simulink model "Form_Finding_Simulink"  (R2022a)
settings: Solver=ode14x  StartTime=0.0  StopTime=0.2  FixedStep=0.00005  RelTol=1e-3
values from neighbouring files (symbols this model uses):
  a_joint = 160/180*pi    (= 2.79252680319)    [Form_Finding_Activation.m]
  F_motor = F    (= 0)    [Form_Finding_Activation.m]
  g = [0;0;-9.81]    [Form_Finding_Activation.m]
  k_cable = 1200    [Form_Finding_Activation.m]
  k_joint = 35    [Form_Finding_Activation.m]
  l_cable = sqrt(6)/4*l_leg*sin(a_joint/2)*(1 - delta)    [Form_Finding_Activation.m]
  m_bar = density*(l_leg*pi*0.005^2)+ m_motor + m_battery    (= 0.662767695314)    [Form_Finding_Activation.m]
  x10_ini = x4_ini+[0 -2*bent_bar 0]    [Form_Finding_Activation.m]
  x11_ini = 2*bent_bar*rotVec([1 0 0],[0 1 0],-90-theta) + x5_ini    [Form_Finding_Activation.m]
  x12_ini = 2*bent_bar*rotVec([1 0 0],[0 1 0],-theta) + x6_ini    [Form_Finding_Activation.m]
  x1_ini = [0 0 0]    [Form_Finding_Activation.m]
  x2_ini = bent_bar*rotVec([1 0 0],[0 1 0],-theta)+ 0.5*sep*rotVec([1 0 0],[0 1 0],90-theta) + [0 sep/2 0]    [Form_Finding_Activation.m]
  x3_ini = [d6x   -sep/2         0]    [Form_Finding_Activation.m]
  x4_ini = bent_bar*rotVec([1 0 0],[0 1 0],-theta) + 0.5*sep*rotVec([1 0 0],[0 1 0],-90-theta) + [0 sep/2 0]    [Form_Finding_Activation.m]
  x5_ini = sep*rotVec([1 0 0],[0 1 0],-theta) + x3_ini    [Form_Finding_Activation.m]
  x6_ini = [0 -sep 0]    [Form_Finding_Activation.m]
  x7_ini = 2*bent_bar*rotVec([1 0 0],[0 1 0],-theta) + x1_ini    [Form_Finding_Activation.m]
  x8_ini = x2_ini + [0 -2*bent_bar 0]    [Form_Finding_Activation.m]
  x9_ini = 2*bent_bar*rotVec([1 0 0],[0 1 0],-90-theta) + x3_ini    [Form_Finding_Activation.m]
undefined symbols (not defined in the file or in its folder): l_bar
(part 1 of 2)
settings Model: Creator=LZY-ALIENWARE15  LastModifiedBy=S2974177
settings SolverCC: ExtrapolationOrder=3  AlgebraicLoopSolver=TrustRegion
settings DebuggingCC: UnconnectedInputMsg=warning  UnconnectedOutputMsg=warning  UnconnectedLineMsg=warning  SFMachineParentedDataDiag=warning
settings RTWCC: DLArmComputeVersion=19.05

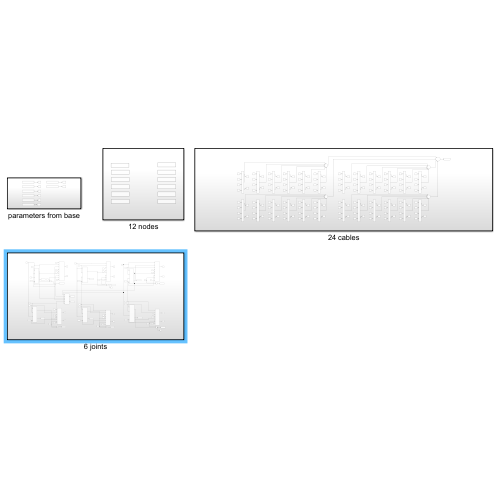
[thumbnail: Simulink's stored preview of the top-level diagram]
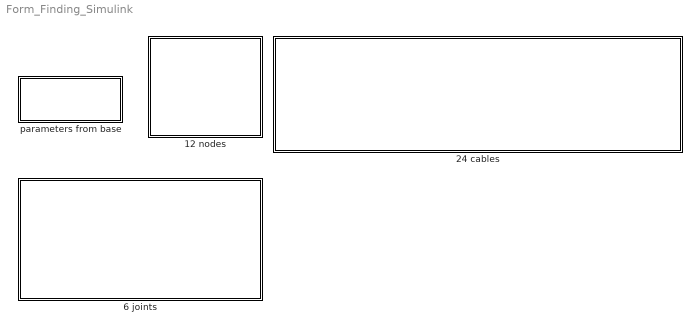
== system Form_Finding_Simulink ==
  "12 nodes " : Subsystem
  24 cables : Subsystem
  6 joints : Subsystem
  parameters from base : Subsystem

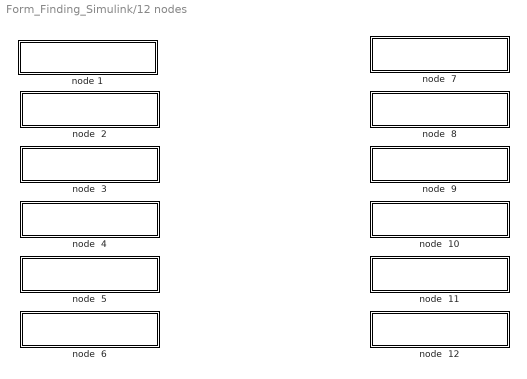
== system Form_Finding_Simulink/12 nodes  ==
  node  10 : Subsystem
  node  11 : Subsystem
  node  12 : Subsystem
  node  2 : Subsystem
  node  3 : Subsystem
  node  4 : Subsystem
  node  5 : Subsystem
  node  6 : Subsystem
  node  7 : Subsystem
  node  8 : Subsystem
  node  9 : Subsystem
  node 1 : Subsystem

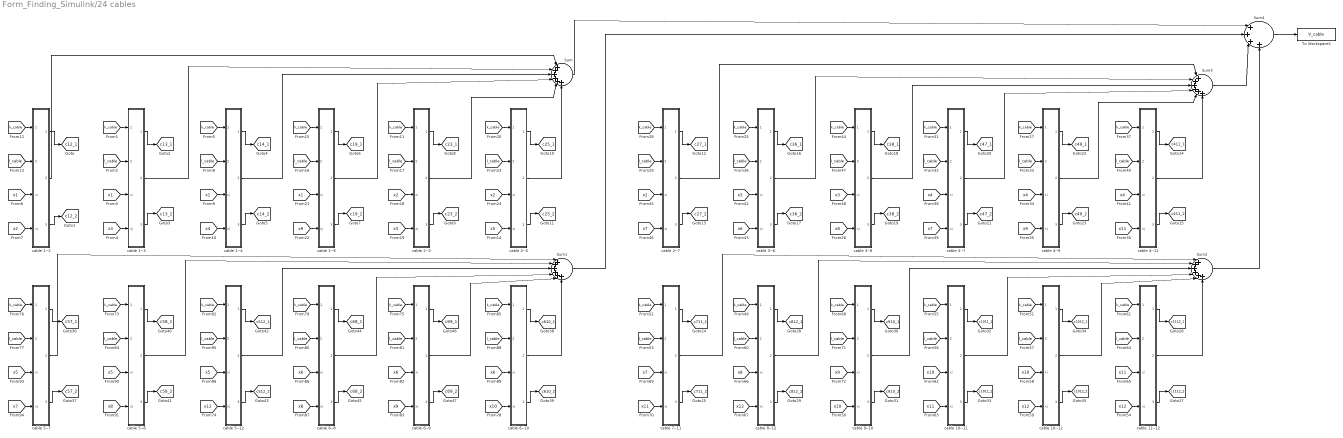
== system Form_Finding_Simulink/24 cables ==
  Sum{,1..3} (4 alike) : Sum  Inputs=|++++++
  Sum4 : Sum  Inputs=|++++
  To Workspace1 : ToWorkspace  VariableName=V_cable  SaveFormat=Timeseries  SampleTime=-1
  cable 1--2 : MATLAB Function  TreatAsAtomicUnit=on
  cable 1--3 : MATLAB Function  TreatAsAtomicUnit=on
  cable 1--4 : MATLAB Function  TreatAsAtomicUnit=on
  cable 1--9 : MATLAB Function  TreatAsAtomicUnit=on
  cable 10--11 : MATLAB Function  TreatAsAtomicUnit=on
  cable 10--12 : MATLAB Function  TreatAsAtomicUnit=on
  cable 11--12 : MATLAB Function  TreatAsAtomicUnit=on
  cable 2--3 : MATLAB Function  TreatAsAtomicUnit=on
  cable 2--5 : MATLAB Function  TreatAsAtomicUnit=on
  cable 2--7 : MATLAB Function  TreatAsAtomicUnit=on
  cable 3--6 : MATLAB Function  TreatAsAtomicUnit=on
  cable 3--8 : MATLAB Function  TreatAsAtomicUnit=on
  cable 4--11 : MATLAB Function  TreatAsAtomicUnit=on
  cable 4--7 : MATLAB Function  TreatAsAtomicUnit=on
  cable 4--9 : MATLAB Function  TreatAsAtomicUnit=on
  cable 5--12 : MATLAB Function  TreatAsAtomicUnit=on
  cable 5--7 : MATLAB Function  TreatAsAtomicUnit=on
  cable 5--8 : MATLAB Function  TreatAsAtomicUnit=on
  cable 6--10 : MATLAB Function  TreatAsAtomicUnit=on
  cable 6--8 : MATLAB Function  TreatAsAtomicUnit=on
  cable 6--9 : MATLAB Function  TreatAsAtomicUnit=on
  cable 7--11 : MATLAB Function  TreatAsAtomicUnit=on
  cable 8--12 : MATLAB Function  TreatAsAtomicUnit=on
  cable 9--10 : MATLAB Function  TreatAsAtomicUnit=on
  tag scope: c1011_1=global, c1011_2=global, c1012_1=global, c1012_2=global, c1112_1=global, c1112_2=global, c12_1=global, c12_2=global, c13_1=global, c13_2=global, c14_1=global, c14_2=global, c19_1=global, c19_2=global, c23_1=global, c23_2=global, c25_1=global, c25_2=global, c27_1=global, c27_2=global, c36_1=global, c36_2=global, c38_1=global, c38_2=global, c411_1=global, c411_2=global, c47_1=global, c47_2=global, c49_1=global, c49_2=global, c512_1=global, c512_2=global, c57_1=global, c57_2=global, c58_1=global, c58_2=global, c610_1=global, c610_2=global, c68_1=global, c68_2=global, c69_1=global, c69_2=global, c711_1=global, c711_2=global, c812_1=global, c812_2=global, c910_1=global, c910_2=global
  wires:
  [k_cable] -> cable 1--2/1(k_cable)
  [x1] -> cable 1--2/3(xi)
  [x2] -> cable 1--2/4(xj)
  cable 1--2/1(out_i) -> [c12_1]
  cable 1--2/3(out_j) -> [c12_2]
  [l_cable] -> cable 1--2/2(l_cable)
  [l_cable] -> cable 1--3/2(l_cable)
  [x1] -> cable 1--3/3(xi)
  [x3] -> cable 1--3/4(xj)
  cable 1--3/3(out_j) -> [c13_2]
  [k_cable] -> cable 1--3/1(k_cable)
  cable 1--3/1(out_i) -> [c13_1]
  [l_cable] -> cable 1--4/2(l_cable)
  [x1] -> cable 1--4/3(xi)
  [x4] -> cable 1--4/4(xj)
  cable 1--4/3(out_j) -> [c14_2]
  [k_cable] -> cable 1--4/1(k_cable)
  cable 1--4/1(out_i) -> [c14_1]
  [l_cable] -> cable 2--3/2(l_cable)
  [k_cable] -> cable 2--5/1(k_cable)
  cable 2--5/1(out_i) -> [c25_1]
  [x2] -> cable 2--5/3(xi)
  cable 2--5/3(out_j) -> [c25_2]
  cable 2--3/1(out_i) -> [c23_1]
  cable 2--3/3(out_j) -> [c23_2]
  [x3] -> cable 2--3/4(xj)
  [x1] -> cable 1--9/3(xi)
  [l_cable] -> cable 1--9/2(l_cable)
  [l_cable] -> cable 2--5/2(l_cable)
  [x9] -> cable 1--9/4(xj)
  [k_cable] -> cable 1--9/1(k_cable)
  [x2] -> cable 2--3/3(xi)
  cable 1--9/3(out_j) -> [c19_2]
  [k_cable] -> cable 2--3/1(k_cable)
  cable 1--9/1(out_i) -> [c19_1]
  [x5] -> cable 2--5/4(xj)
  [l_cable] -> cable 3--6/2(l_cable)
  [k_cable] -> cable 3--8/1(k_cable)
  cable 3--8/1(out_i) -> [c38_1]
  cable 3--8/3(out_j) -> [c38_2]
  cable 3--6/1(out_i) -> [c36_1]
  cable 3--6/3(out_j) -> [c36_2]
  [x6] -> cable 3--6/4(xj)
  [x7] -> cable 4--7/4(xj)
  [l_cable] -> cable 4--7/2(l_cable)
  [x4] -> cable 4--7/3(xi)
  [x9] -> cable 4--9/4(xj)
  cable 4--9/3(out_j) -> [c49_2]
  cable 4--11/3(out_j) -> [c411_2]
  [x4] -> cable 4--11/3(xi)
  [x11] -> cable 4--11/4(xj)
  cable 4--9/1(out_i) -> [c49_1]
  cable 4--7/1(out_i) -> [c47_1]
  [k_cable] -> cable 4--9/1(k_cable)
  cable 4--7/3(out_j) -> [c47_2]
  [k_cable] -> cable 4--7/1(k_cable)
  [x4] -> cable 4--9/3(xi)
  [x7] -> cable 2--7/4(xj)
  cable 2--7/3(out_j) -> [c27_2]
  [x3] -> cable 3--6/3(xi)
  [k_cable] -> cable 2--7/1(k_cable)
  [l_cable] -> cable 4--11/2(l_cable)
  cable 4--11/1(out_i) -> [c411_1]
  [x3] -> cable 3--8/3(xi)
  cable 2--7/1(out_i) -> [c27_1]
  [k_cable] -> cable 3--6/1(k_cable)
  [x8] -> cable 3--8/4(xj)
  [k_cable] -> cable 4--11/1(k_cable)
  [x2] -> cable 2--7/3(xi)
  [l_cable] -> cable 2--7/2(l_cable)
  [l_cable] -> cable 3--8/2(l_cable)
  [l_cable] -> cable 4--9/2(l_cable)
  [l_cable] -> cable 8--12/2(l_cable)
  [k_cable] -> cable 9--10/1(k_cable)
  cable 9--10/1(out_i) -> [c910_1]
  cable 9--10/3(out_j) -> [c910_2]
  cable 8--12/1(out_i) -> [c812_1]
  cable 8--12/3(out_j) -> [c812_2]
  [x12] -> cable 8--12/4(xj)
  [x11] -> cable 10--11/4(xj)
  [l_cable] -> cable 10--11/2(l_cable)
  [x10] -> cable 10--11/3(xi)
  [x12] -> cable 10--12/4(xj)
  cable 10--12/3(out_j) -> [c1012_2]
  cable 11--12/3(out_j) -> [c1112_2]
  [x11] -> cable 11--12/3(xi)
  [x12] -> cable 11--12/4(xj)
  cable 10--12/1(out_i) -> [c1012_1]
  cable 10--11/1(out_i) -> [c1011_1]
  [k_cable] -> cable 10--12/1(k_cable)
  cable 10--11/3(out_j) -> [c1011_2]
  [k_cable] -> cable 10--11/1(k_cable)
  [x10] -> cable 10--12/3(xi)
  [x11] -> cable 7--11/4(xj)
  cable 7--11/3(out_j) -> [c711_2]
  [x8] -> cable 8--12/3(xi)
  [k_cable] -> cable 7--11/1(k_cable)
  [l_cable] -> cable 11--12/2(l_cable)
  cable 11--12/1(out_i) -> [c1112_1]
  [x9] -> cable 9--10/3(xi)
  cable 7--11/1(out_i) -> [c711_1]
  [k_cable] -> cable 8--12/1(k_cable)
  [x10] -> cable 9--10/4(xj)
  [k_cable] -> cable 11--12/1(k_cable)
  [x7] -> cable 7--11/3(xi)
  [l_cable] -> cable 7--11/2(l_cable)
  [l_cable] -> cable 9--10/2(l_cable)
  [l_cable] -> cable 10--12/2(l_cable)
  [l_cable] -> cable 5--8/2(l_cable)
  [k_cable] -> cable 5--12/1(k_cable)
  cable 5--12/1(out_i) -> [c512_1]
  cable 5--12/3(out_j) -> [c512_2]
  cable 5--8/1(out_i) -> [c58_1]
  cable 5--8/3(out_j) -> [c58_2]
  [x8] -> cable 5--8/4(xj)
  [x8] -> cable 6--8/4(xj)
  [l_cable] -> cable 6--8/2(l_cable)
  [x6] -> cable 6--8/3(xi)
  [x9] -> cable 6--9/4(xj)
  cable 6--9/3(out_j) -> [c69_2]
  cable 6--10/3(out_j) -> [c610_2]
  [x6] -> cable 6--10/3(xi)
  [x10] -> cable 6--10/4(xj)
  cable 6--9/1(out_i) -> [c69_1]
  cable 6--8/1(out_i) -> [c68_1]
  [k_cable] -> cable 6--9/1(k_cable)
  cable 6--8/3(out_j) -> [c68_2]
  [k_cable] -> cable 6--8/1(k_cable)
  [x6] -> cable 6--9/3(xi)
  [x7] -> cable 5--7/4(xj)
  cable 5--7/3(out_j) -> [c57_2]
  [x5] -> cable 5--8/3(xi)
  [k_cable] -> cable 5--7/1(k_cable)
  [l_cable] -> cable 6--10/2(l_cable)
  cable 6--10/1(out_i) -> [c610_1]
  [x5] -> cable 5--12/3(xi)
  cable 5--7/1(out_i) -> [c57_1]
  [k_cable] -> cable 5--8/1(k_cable)
  [x12] -> cable 5--12/4(xj)
  [k_cable] -> cable 6--10/1(k_cable)
  [x5] -> cable 5--7/3(xi)
  [l_cable] -> cable 5--7/2(l_cable)
  [l_cable] -> cable 5--12/2(l_cable)
  [l_cable] -> cable 6--9/2(l_cable)
  cable 1--2/2(E_cable) -> Sum/1
  cable 10--11/2(E_cable) -> Sum2/4
  cable 9--10/2(E_cable) -> Sum2/3
  cable 10--12/2(E_cable) -> Sum2/5
  cable 11--12/2(E_cable) -> Sum2/6
  cable 8--12/2(E_cable) -> Sum2/2
  cable 7--11/2(E_cable) -> Sum2/1
  cable 6--10/2(E_cable) -> Sum1/6
  cable 6--9/2(E_cable) -> Sum1/5
  cable 6--8/2(E_cable) -> Sum1/4
  cable 5--12/2(E_cable) -> Sum1/3
  cable 5--8/2(E_cable) -> Sum1/2
  cable 5--7/2(E_cable) -> Sum1/1
  cable 1--3/2(E_cable) -> Sum/2
  cable 1--4/2(E_cable) -> Sum/3
  cable 1--9/2(E_cable) -> Sum/4
  cable 2--3/2(E_cable) -> Sum/5
  cable 2--5/2(E_cable) -> Sum/6
  cable 2--7/2(E_cable) -> Sum3/1
  cable 3--6/2(E_cable) -> Sum3/2
  cable 3--8/2(E_cable) -> Sum3/3
  cable 4--7/2(E_cable) -> Sum3/4
  cable 4--9/2(E_cable) -> Sum3/5
  cable 4--11/2(E_cable) -> Sum3/6
  Sum3/1 -> Sum4/3
  Sum2/1 -> Sum4/4
  Sum1/1 -> Sum4/2
  Sum/1 -> Sum4/1
  Sum4/1 -> To Workspace1/1

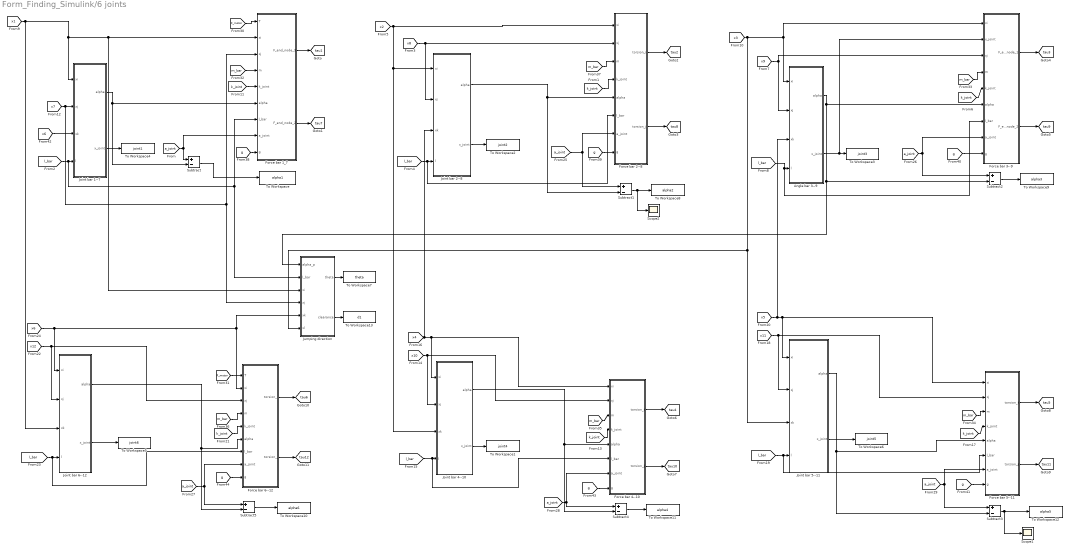
== system Form_Finding_Simulink/6 joints ==
  Angle bar 3--9 : MATLAB Function  TreatAsAtomicUnit=on
  Force bar 1_7 : MATLAB Function  TreatAsAtomicUnit=on
  Force bar 2--8 : MATLAB Function  TreatAsAtomicUnit=on
  Force bar 3--9 : MATLAB Function  TreatAsAtomicUnit=on
  Force bar 4--10 : MATLAB Function  TreatAsAtomicUnit=on
  Force bar 5--11 : MATLAB Function  TreatAsAtomicUnit=on
  Force bar 6--12 : MATLAB Function  TreatAsAtomicUnit=on
  Joint bar 1--7 : MATLAB Function  TreatAsAtomicUnit=on
  Joint bar 2--8 : MATLAB Function  TreatAsAtomicUnit=on
  Joint bar 4--10 : MATLAB Function  TreatAsAtomicUnit=on
  Joint bar 5--11 : MATLAB Function  TreatAsAtomicUnit=on
  Joint bar 6--12 : MATLAB Function  TreatAsAtomicUnit=on
  Jumping direction : MATLAB Function  TreatAsAtomicUnit=on
  Scope1 : Scope
  Scope2 : Scope
  Subtract{,1..5} (6 alike) : Sum  Inputs=+-
  To Workspace : ToWorkspace  VariableName=alpha1  SaveFormat=Timeseries  SampleTime=-1
  To Workspace1 : ToWorkspace  VariableName=joint4  SaveFormat=Timeseries  SampleTime=-1
  To Workspace10 : ToWorkspace  VariableName=alpha6  SaveFormat=Timeseries  SampleTime=-1
  To Workspace11 : ToWorkspace  VariableName=alpha4  SaveFormat=Timeseries  SampleTime=-1
  To Workspace12 : ToWorkspace  VariableName=alpha5  SaveFormat=Timeseries  SampleTime=-1
  To Workspace13 : ToWorkspace  VariableName=d1  SaveFormat=Timeseries  SampleTime=-1
  To Workspace2 : ToWorkspace  VariableName=joint2  SaveFormat=Timeseries  SampleTime=-1
  To Workspace3 : ToWorkspace  VariableName=joint3  SaveFormat=Timeseries  SampleTime=-1
  To Workspace4 : ToWorkspace  VariableName=joint1  SaveFormat=Timeseries  SampleTime=-1
  To Workspace5 : ToWorkspace  VariableName=joint6  SaveFormat=Timeseries  SampleTime=-1
  To Workspace6 : ToWorkspace  VariableName=joint5  SaveFormat=Timeseries  SampleTime=-1
  To Workspace7 : ToWorkspace  VariableName=theta  SaveFormat=Timeseries  SampleTime=-1
  To Workspace8 : ToWorkspace  VariableName=alpha2  SaveFormat=Timeseries  SampleTime=-1
  To Workspace9 : ToWorkspace  VariableName=alpha3  SaveFormat=Timeseries  SampleTime=-1
  tag scope: tau10=global, tau11=global, tau12=global, tau1=global, tau2=global, tau3=global, tau4=global, tau5=global, tau6=global, tau7=global, tau8=global, tau9=global
  wires:
  [x1] -> Joint bar 1--7/1(xi), Jumping direction/3(xi), Force bar 1_7/2(xi), Joint bar 6--12/3(xk)
  [x7] -> Jumping direction/4(xj), Force bar 1_7/3(xj), Joint bar 1--7/2(xj)
  Joint bar 1--7/1(alpha) -> Subtract/2, Force bar 1_7/6(alpha)
  Force bar 1_7/1(F_end_node_1) -> [tau1]
  [k_joint] -> Force bar 1_7/5(k_joint)
  [l_bar] -> Jumping direction/2(l_bar), Force bar 1_7/7(l_bar), Joint bar 1--7/4(l)
  Force bar 2--8/2(torsion_j) -> [tau8]
  [x2] -> Joint bar 2--8/1(xi), Joint bar 4--10/3(xk), Force bar 2--8/1(xi)
  [k_joint] -> Force bar 2--8/4(k_joint)
  [l_bar] -> Force bar 2--8/6(l_bar), Joint bar 2--8/4(l)
  Force bar 2--8/1(torsion_i) -> [tau2]
  [x8] -> Joint bar 2--8/2(xj), Force bar 2--8/2(xj)
  [l_bar] -> Force bar 3--9/7(l_bar), Angle bar 3--9/4(l)
  Force bar 3--9/2(F_end_node_2) -> [tau9]
  Force bar 3--9/1(F_end_node_1) -> [tau3]
  [x3] -> Jumping direction/6(xl), Joint bar 5--11/3(xk), Force bar 3--9/1(xi), Angle bar 3--9/1(xi)
  [k_joint] -> Force bar 3--9/5(k_joint)
  [x9] -> Force bar 3--9/3(xj), Angle bar 3--9/2(xj)
  [x10] -> Force bar 4--10/2(xj), Joint bar 4--10/2(xj)
  Force bar 4--10/2(torsion_j) -> [tau10]
  [x4] -> Joint bar 4--10/1(xi), Force bar 4--10/1(xi), Joint bar 2--8/3(xk)
  [k_joint] -> Force bar 4--10/4(k_joint)
  [l_bar] -> Force bar 4--10/6(l_bar), Joint bar 4--10/4(l)
  Force bar 4--10/1(torsion_i) -> [tau4]
  [l_bar] -> Force bar 5--11/6(l_bar), Joint bar 5--11/4(l)
  [k_joint] -> Force bar 5--11/4(k_joint)
  Force bar 5--11/1(torsion_i) -> [tau5]
  [x5] -> Angle bar 3--9/3(xk), Joint bar 5--11/1(xi), Force bar 5--11/1(xi)
  Force bar 5--11/2(torsion_j) -> [tau11]
  [x12] -> Joint bar 6--12/2(xj), Force bar 6--12/3(xj)
  [k_joint] -> Force bar 6--12/5(k_joint)
  Force bar 6--12/1(torsion_i) -> [tau6]
  [x6] -> Jumping direction/5(xk), Force bar 6--12/2(xi), Joint bar 6--12/1(xi)
  Force bar 6--12/2(torsion_j) -> [tau12]
  [a_joint] -> Subtract/1, Force bar 1_7/8(a_joint)
  [a_joint] -> Force bar 6--12/8(a_joint), Subtract5/1
  [x11] -> Joint bar 5--11/2(xj), Force bar 5--11/2(xj)
  [F_motor] -> Force bar 1_7/1(T)
  [F_motor] -> Force bar 6--12/1(T)
  Jumping direction/1(theta) -> To Workspace7/1
  Jumping direction/2(clearance) -> To Workspace13/1
  Joint bar 2--8/1(alpha) -> Subtract1/2, Force bar 2--8/5(alpha)
  [a_joint] -> Subtract1/1, Force bar 2--8/7(a_joint)
  Subtract1/1 -> To Workspace8/1, Scope2/1
  Angle bar 3--9/1(alpha) -> Subtract2/2, Jumping direction/1(alpha_p), Force bar 3--9/6(alpha)
  [a_joint] -> Force bar 3--9/8(a_joint), Subtract2/1
  Subtract2/1 -> To Workspace9/1
  Joint bar 5--11/1(alpha) -> Subtract3/2, Force bar 5--11/5(alpha)
  [a_joint] -> Force bar 5--11/7(a_joint), Subtract3/1
  Subtract3/1 -> Scope1/1, To Workspace12/1
  Joint bar 4--10/1(alpha) -> Subtract4/2, Force bar 4--10/5(alpha)
  [a_joint] -> Subtract4/1, Force bar 4--10/7(a_joint)
  Subtract4/1 -> To Workspace11/1
  Joint bar 6--12/1(alpha) -> Subtract5/2, Force bar 6--12/6(alpha)
  [l_bar] -> Force bar 6--12/7(l_bar), Joint bar 6--12/4(l)
  Subtract5/1 -> To Workspace10/1
  [m_bar] -> Force bar 1_7/4(m)
  Force bar 1_7/2(F_end_node_2) -> [tau7]
  [m_bar] -> Force bar 3--9/4(m)
  [m_bar] -> Force bar 5--11/3(m)
  [m_bar] -> Force bar 4--10/3(m)
  [m_bar] -> Force bar 6--12/4(m)
  [m_bar] -> Force bar 2--8/3(m)
  Subtract/1 -> To Workspace/1
  Joint bar 2--8/2(x_joint) -> To Workspace2/1
  Joint bar 5--11/2(x_joint) -> To Workspace6/1
  Joint bar 4--10/2(x_joint) -> To Workspace1/1
  Joint bar 6--12/2(x_joint) -> To Workspace5/1
  Angle bar 3--9/2(x_joint) -> Force bar 3--9/2(x_joint), To Workspace3/1
  Joint bar 1--7/2(x_joint) -> To Workspace4/1
  [x6] -> Joint bar 1--7/3(xk)
  [g] -> Force bar 1_7/9(g)
  [g] -> Force bar 2--8/8(g)
  [g] -> Force bar 3--9/9(g)
  [g] -> Force bar 5--11/8(g)
  [g] -> Force bar 4--10/8(g)
  [g] -> Force bar 6--12/9(g)

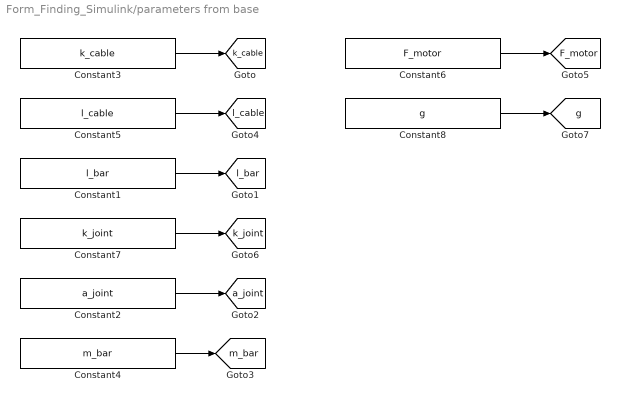
== system Form_Finding_Simulink/parameters from base ==
  Constant1 : Constant  Value=l_bar
  Constant2 : Constant  Value=a_joint
  Constant3 : Constant  Value=k_cable
  Constant4 : Constant  Value=m_bar
  Constant5 : Constant  Value=l_cable
  Constant6 : Constant  Value=F_motor
  Constant7 : Constant  Value=k_joint
  Constant8 : Constant  Value=g
  tag scope: F_motor=global, a_joint=global, g=global, k_cable=global, k_joint=global, l_bar=global, l_cable=global, m_bar=global
  wires:
  Constant3/1 -> [k_cable]
  Constant1/1 -> [l_bar]
  Constant5/1 -> [l_cable]
  Constant7/1 -> [k_joint]
  Constant2/1 -> [a_joint]
  Constant6/1 -> [F_motor]
  Constant4/1 -> [m_bar]
  Constant8/1 -> [g]

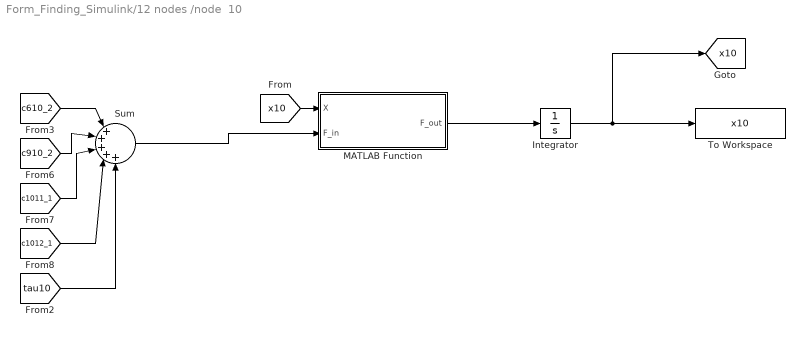
== system Form_Finding_Simulink/12 nodes /node  10 ==
  Integrator : Integrator  InitialCondition=x10_ini  UpperSaturationLimit=2  LowerSaturationLimit=-2
  MATLAB Function : MATLAB Function  TreatAsAtomicUnit=on
  Sum : Sum  Inputs=|+++++
  To Workspace : ToWorkspace  VariableName=x10  SaveFormat=Timeseries  SampleTime=-1
  tag scope: x10=global
  wires:
  Integrator/1 -> [x10], To Workspace/1
  [c910_2] -> Sum/2
  [c1011_1] -> Sum/3
  [c1012_1] -> Sum/4
  [c610_2] -> Sum/1
  [tau10] -> Sum/5
  [x10] -> MATLAB Function/1(X)
  MATLAB Function/1(F_out) -> Integrator/1
  Sum/1 -> MATLAB Function/2(F_in)

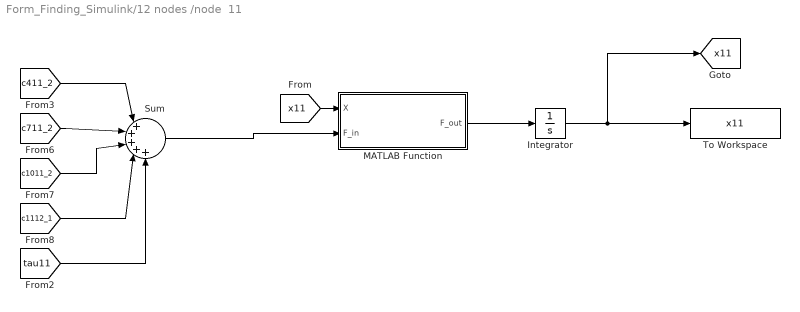
== system Form_Finding_Simulink/12 nodes /node  11 ==
  Integrator : Integrator  InitialCondition=x11_ini  UpperSaturationLimit=2  LowerSaturationLimit=-2
  MATLAB Function : MATLAB Function  TreatAsAtomicUnit=on
  Sum : Sum  Inputs=|+++++
  To Workspace : ToWorkspace  VariableName=x11  SaveFormat=Timeseries  SampleTime=-1
  tag scope: x11=global
  wires:
  Integrator/1 -> [x11], To Workspace/1
  [c711_2] -> Sum/2
  [c1011_2] -> Sum/3
  [c1112_1] -> Sum/4
  [c411_2] -> Sum/1
  [tau11] -> Sum/5
  [x11] -> MATLAB Function/1(X)
  MATLAB Function/1(F_out) -> Integrator/1
  Sum/1 -> MATLAB Function/2(F_in)

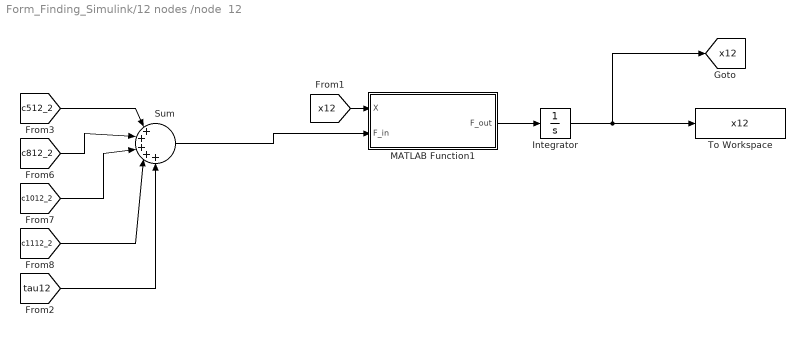
== system Form_Finding_Simulink/12 nodes /node  12 ==
  Integrator : Integrator  InitialCondition=x12_ini  UpperSaturationLimit=2  LowerSaturationLimit=-2
  MATLAB Function1 : MATLAB Function  TreatAsAtomicUnit=on
  Sum : Sum  Inputs=|+++++
  To Workspace : ToWorkspace  VariableName=x12  SaveFormat=Timeseries  SampleTime=-1
  tag scope: x12=global
  wires:
  Integrator/1 -> [x12], To Workspace/1
  [c812_2] -> Sum/2
  [c1012_2] -> Sum/3
  [c1112_2] -> Sum/4
  [c512_2] -> Sum/1
  [tau12] -> Sum/5
  [x12] -> MATLAB Function1/1(X)
  MATLAB Function1/1(F_out) -> Integrator/1
  Sum/1 -> MATLAB Function1/2(F_in)

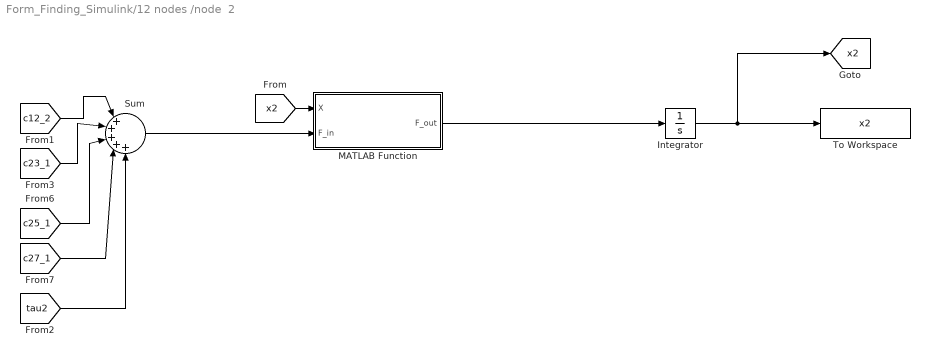
== system Form_Finding_Simulink/12 nodes /node  2 ==
  Integrator : Integrator  InitialCondition=x2_ini  UpperSaturationLimit=2  LowerSaturationLimit=-2
  MATLAB Function : MATLAB Function  TreatAsAtomicUnit=on
  Sum : Sum  Inputs=|+++++
  To Workspace : ToWorkspace  VariableName=x2  SaveFormat=Timeseries  SampleTime=-1
  tag scope: x2=global
  wires:
  Integrator/1 -> [x2], To Workspace/1
  Sum/1 -> MATLAB Function/2(F_in)
  [c12_2] -> Sum/1
  [c23_1] -> Sum/2
  [c27_1] -> Sum/4
  [c25_1] -> Sum/3
  [tau2] -> Sum/5
  MATLAB Function/1(F_out) -> Integrator/1
  [x2] -> MATLAB Function/1(X)

== system Form_Finding_Simulink/12 nodes /node  3 ==
  Integrator : Integrator  InitialCondition=x3_ini  UpperSaturationLimit=2  LowerSaturationLimit=-2
  Sum : Sum  Inputs=|+++++
  To Workspace : ToWorkspace  VariableName=x3  SaveFormat=Timeseries  SampleTime=-1
  node 1 constrain : MATLAB Function  TreatAsAtomicUnit=on
  tag scope: x3=global
  wires:
  Integrator/1 -> [x3], To Workspace/1
  [c38_1] -> Sum/4
  [c23_2] -> Sum/2
  [c36_1] -> Sum/3
  [c13_2] -> Sum/1
  [tau3] -> Sum/5
  node 1 constrain/1(control_out) -> Integrator/1
  Sum/1 -> node 1 constrain/1(control_in)

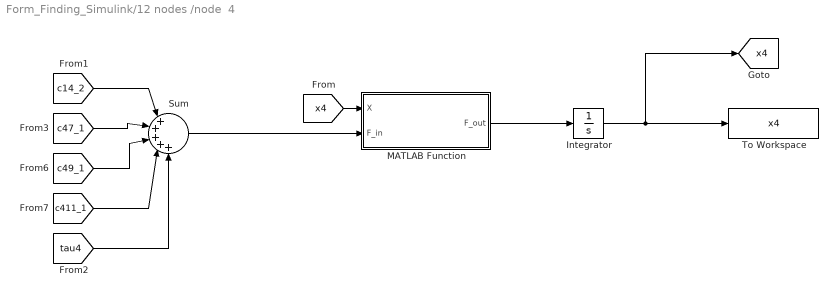
== system Form_Finding_Simulink/12 nodes /node  4 ==
  Integrator : Integrator  InitialCondition=x4_ini  UpperSaturationLimit=2  LowerSaturationLimit=-2
  MATLAB Function : MATLAB Function  TreatAsAtomicUnit=on
  Sum : Sum  Inputs=|+++++
  To Workspace : ToWorkspace  VariableName=x4  SaveFormat=Timeseries  SampleTime=-1
  tag scope: x4=global
  wires:
  Integrator/1 -> [x4], To Workspace/1
  [c411_1] -> Sum/4
  [c47_1] -> Sum/2
  [c49_1] -> Sum/3
  [c14_2] -> Sum/1
  [tau4] -> Sum/5
  [x4] -> MATLAB Function/1(X)
  MATLAB Function/1(F_out) -> Integrator/1
  Sum/1 -> MATLAB Function/2(F_in)

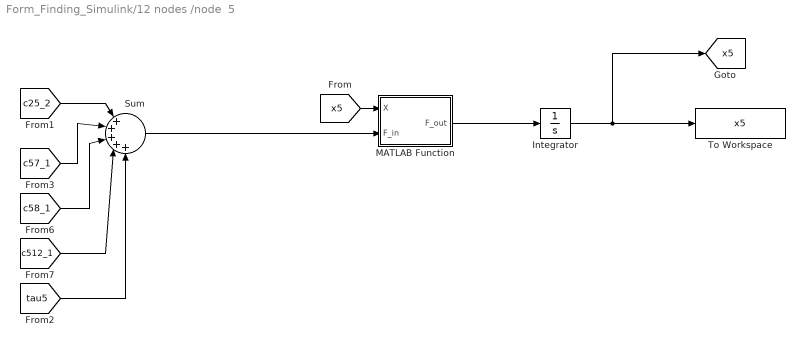
== system Form_Finding_Simulink/12 nodes /node  5 ==
  Integrator : Integrator  InitialCondition=x5_ini  UpperSaturationLimit=2  LowerSaturationLimit=-2
  MATLAB Function : MATLAB Function  TreatAsAtomicUnit=on
  Sum : Sum  Inputs=|+++++
  To Workspace : ToWorkspace  VariableName=x5  SaveFormat=Timeseries  SampleTime=-1
  tag scope: x5=global
  wires:
  Integrator/1 -> [x5], To Workspace/1
  [c57_1] -> Sum/2
  [c58_1] -> Sum/3
  [c512_1] -> Sum/4
  [c25_2] -> Sum/1
  Sum/1 -> MATLAB Function/2(F_in)
  [tau5] -> Sum/5
  MATLAB Function/1(F_out) -> Integrator/1
  [x5] -> MATLAB Function/1(X)

== system Form_Finding_Simulink/12 nodes /node  6 ==
  Integrator : Integrator  InitialCondition=x6_ini  UpperSaturationLimit=2  LowerSaturationLimit=-2
  Sum : Sum  Inputs=|+++++
  To Workspace : ToWorkspace  VariableName=x6  SaveFormat=Timeseries  SampleTime=-1
  node 6 constrain1 : MATLAB Function  TreatAsAtomicUnit=on
  tag scope: x6=global
  wires:
  Integrator/1 -> [x6], To Workspace/1
  [c68_1] -> Sum/2
  [c69_1] -> Sum/3
  [c610_1] -> Sum/4
  [c36_2] -> Sum/1
  [tau6] -> Sum/5
  node 6 constrain1/1(control_out) -> Integrator/1
  Sum/1 -> node 6 constrain1/1(control_in)

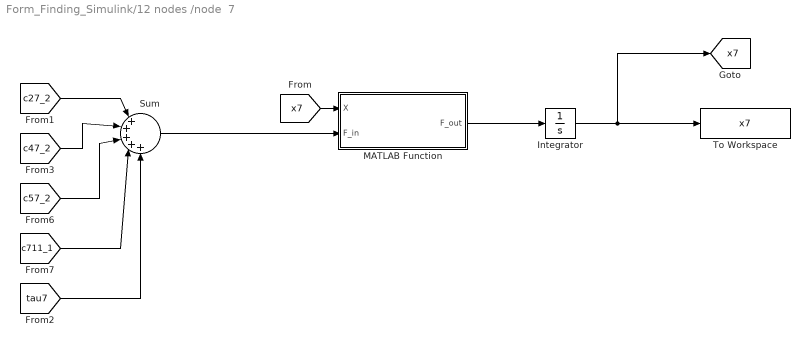
== system Form_Finding_Simulink/12 nodes /node  7 ==
  Integrator : Integrator  InitialCondition=x7_ini  UpperSaturationLimit=2  LowerSaturationLimit=-2
  MATLAB Function : MATLAB Function  TreatAsAtomicUnit=on
  Sum : Sum  Inputs=|+++++
  To Workspace : ToWorkspace  VariableName=x7  SaveFormat=Timeseries  SampleTime=-1
  tag scope: x7=global
  wires:
  Integrator/1 -> [x7], To Workspace/1
  [c47_2] -> Sum/2
  [c57_2] -> Sum/3
  [c711_1] -> Sum/4
  [c27_2] -> Sum/1
  [tau7] -> Sum/5
  [x7] -> MATLAB Function/1(X)
  MATLAB Function/1(F_out) -> Integrator/1
  Sum/1 -> MATLAB Function/2(F_in)

== system Form_Finding_Simulink/12 nodes /node  8 ==
  Integrator : Integrator  InitialCondition=x8_ini  UpperSaturationLimit=2  LowerSaturationLimit=-2
  MATLAB Function : MATLAB Function  TreatAsAtomicUnit=on
  Sum : Sum  Inputs=|+++++
  To Workspace : ToWorkspace  VariableName=x8  SaveFormat=Timeseries  SampleTime=-1
  tag scope: x8=global
  wires:
  Integrator/1 -> [x8], To Workspace/1
  [c58_2] -> Sum/2
  [c68_2] -> Sum/3
  [c812_1] -> Sum/4
  [c38_2] -> Sum/1
  [tau8] -> Sum/5
  [x8] -> MATLAB Function/1(X)
  MATLAB Function/1(F_out) -> Integrator/1
  Sum/1 -> MATLAB Function/2(F_in)

== system Form_Finding_Simulink/12 nodes /node  9 ==
  Integrator : Integrator  InitialCondition=x9_ini  UpperSaturationLimit=2  LowerSaturationLimit=-2
  MATLAB Function : MATLAB Function  TreatAsAtomicUnit=on
  Sum : Sum  Inputs=|+++++
  To Workspace : ToWorkspace  VariableName=x9  SaveFormat=Timeseries  SampleTime=-1
  tag scope: x9=global
  wires:
  Integrator/1 -> [x9], To Workspace/1
  [c49_2] -> Sum/2
  [c69_2] -> Sum/3
  [c910_1] -> Sum/4
  [c19_2] -> Sum/1
  [tau9] -> Sum/5
  [x9] -> MATLAB Function/1(X)
  MATLAB Function/1(F_out) -> Integrator/1
  Sum/1 -> MATLAB Function/2(F_in)

== system Form_Finding_Simulink/12 nodes /node 1 ==
  Integrator : Integrator  InitialCondition=x1_ini  UpperSaturationLimit=2  LowerSaturationLimit=-2
  Sum : Sum  Inputs=|+++++
  To Workspace : ToWorkspace  VariableName=x1  SaveFormat=Timeseries  SampleTime=-1
  node 1 constrain : MATLAB Function  TreatAsAtomicUnit=on
  tag scope: x1=global
  wires:
  Integrator/1 -> [x1], To Workspace/1
  [c12_1] -> Sum/1
  [c13_1] -> Sum/2
  [c14_1] -> Sum/3
  [c19_1] -> Sum/4
  [tau1] -> Sum/5
  node 1 constrain/1(control_out) -> Integrator/1
  Sum/1 -> node 1 constrain/1(control_in)

== matlab function Form_Finding_Simulink/6 joints/Joint bar 1--7 ==
  data: xi input; alpha output; xj input; xk input; l input; x_joint output
function [alpha, x_joint]  = angle(xi, xj, xk, l)
%% Calculating the angle
d = norm(xi - xj); % Nodal distance
mag = (l^2-2*d^2)/l^2; % Term inside the inverse cosine to calculate the angle
alpha = acos(mag); % Angle of the joint

%% Plotting the Joint
% Distance from axis
d = l/2*cos(alpha/2);

% Vectors used for determination of the normal vector
nxi = transpose(xi);
nxj = transpose(xj);
nxk = transpose(xk);

% Normal vector of a plane created by a set of 2 parallel bars
normal = cross(nxi-nxj, nxi-nxk);
N = normal/norm(normal);

% Vector along the line between bar-connected nodes
x = nxj - nxi;
X = x/norm(x);

% Vector pointing outwards 
V = rotVec(X,N,-90);

% Position vector of the joint, to be used for plotting
x_joint = transpose(d*V + (nxj+nxi)/2);

end

== matlab function Form_Finding_Simulink/6 joints/Force bar 1_7 ==
  data: T input; F_end_node_1 output; xi input; xj input; m input; k_joint input; alpha input; l_bar input; a_joint input; F_end_node_2 output; g input
function [F_end_node_1, F_end_node_2]= Force(T, xi, xj, m, k_joint, alpha, l_bar, a_joint, g)
% Node distance
dist = norm(xj-xi);

% Force exerted by the joint at the end node. The force is zero when the
% deflection angle is larger than a_joint
if alpha < a_joint
    F_torsion = 1/2 * k_joint * (a_joint - alpha) / (cos(alpha/2)*l_bar/2);
else
    F_torsion = 0;
end

% Gravitational force
Fg_j = m*g/2;

% Motor Force, also with the lever effect incorporated
F_motor = T/(l_bar*cos(alpha/2)); % T is in [N m]

% Calculation of the two parts of the torsion
F_end_node_1 = (F_torsion - F_motor) *(xi-xj)/dist; % No gravity on this node because it is on the ground
F_end_node_2 = (F_torsion - F_motor) *(xj-xi)/dist + Fg_j;

end

== matlab function Form_Finding_Simulink/12 nodes /node  5/MATLAB Function ==
  data: X input; F_out output; F_in input
function F_out = ground_constraint(X,F_in)
if X(3) <= 0 && F_in(3) < 0 
    F_out = [F_in(1);F_in(2);0];
else
    F_out = F_in;
end
end

== matlab function Form_Finding_Simulink/12 nodes /node  2/MATLAB Function ==
  data: X input; F_out output; F_in input
function F_out = ground_constraint(X,F_in)
if X(3) <= 0 && F_in(3) < 0 
    F_out = [F_in(1);F_in(2);0];
else
    F_out = F_in;
end
end

== matlab function Form_Finding_Simulink/24 cables/cable 1--9 ==
  data: out_i output; E_cable output; out_j output; k_cable input; l_cable input; xi input; xj input
function [out_i, E_cable, out_j]= cable(k_cable, l_cable,xi,xj)
% Node distance
dist = norm(xi-xj);

% Difference of node distance with the cable rest length
D = dist-l_cable;

% If the cable is in tension, then the force is calculated. When the cable is slack, the force is zero 
if  dist-l_cable >= 0
    D = dist-l_cable;
elseif dist-l_cable < 0
    D = 0;
end

% Forces on end nodes
out_i = k_cable*D*(xj-xi)/dist;
out_j = -k_cable*D*(xj-xi)/dist;

% Potential energy stored in the cable
E_cable = 0.5*k_cable*D^2;
end

== matlab function Form_Finding_Simulink/24 cables/cable 2--5 ==
  data: out_i output; E_cable output; out_j output; k_cable input; l_cable input; xi input; xj input
function [out_i, E_cable, out_j]= cable(k_cable, l_cable,xi,xj)
% Node distance
dist = norm(xi-xj);

% Difference of node distance with the cable rest length
D = dist-l_cable;

% If the cable is in tension, then the force is calculated. When the cable is slack, the force is zero 
if  dist-l_cable >= 0
    D = dist-l_cable;
elseif dist-l_cable < 0
    D = 0;
end

% Forces on end nodes
out_i = k_cable*D*(xj-xi)/dist;
out_j = -k_cable*D*(xj-xi)/dist;

% Potential energy stored in the cable
E_cable = 0.5*k_cable*D^2;
end

== matlab function Form_Finding_Simulink/24 cables/cable 4--9 ==
  data: out_i output; E_cable output; out_j output; k_cable input; l_cable input; xi input; xj input
function [out_i, E_cable, out_j]= cable(k_cable, l_cable,xi,xj)
% Node distance
dist = norm(xi-xj);

% Difference of node distance with the cable rest length
D = dist-l_cable;

% If the cable is in tension, then the force is calculated. When the cable is slack, the force is zero 
if  dist-l_cable >= 0
    D = dist-l_cable;
elseif dist-l_cable < 0
    D = 0;
end

% Forces on end nodes
out_i = k_cable*D*(xj-xi)/dist;
out_j = -k_cable*D*(xj-xi)/dist;

% Potential energy stored in the cable
E_cable = 0.5*k_cable*D^2;
end

== matlab function Form_Finding_Simulink/24 cables/cable 4--7 ==
  data: out_i output; E_cable output; out_j output; k_cable input; l_cable input; xi input; xj input
function [out_i, E_cable, out_j]= cable(k_cable, l_cable,xi,xj)
% Node distance
dist = norm(xi-xj);

% Difference of node distance with the cable rest length
D = dist-l_cable;

% If the cable is in tension, then the force is calculated. When the cable is slack, the force is zero 
if  dist-l_cable >= 0
    D = dist-l_cable;
elseif dist-l_cable < 0
    D = 0;
end

% Forces on end nodes
out_i = k_cable*D*(xj-xi)/dist;
out_j = -k_cable*D*(xj-xi)/dist;

% Potential energy stored in the cable
E_cable = 0.5*k_cable*D^2;
end

== matlab function Form_Finding_Simulink/24 cables/cable 4--11 ==
  data: out_i output; E_cable output; out_j output; k_cable input; l_cable input; xi input; xj input
function [out_i, E_cable, out_j]= cable(k_cable, l_cable,xi,xj)
% Node distance
dist = norm(xi-xj);

% Difference of node distance with the cable rest length
D = dist-l_cable;

% If the cable is in tension, then the force is calculated. When the cable is slack, the force is zero 
if  dist-l_cable >= 0
    D = dist-l_cable;
elseif dist-l_cable < 0
    D = 0;
end

% Forces on end nodes
out_i = k_cable*D*(xj-xi)/dist;
out_j = -k_cable*D*(xj-xi)/dist;

% Potential energy stored in the cable
E_cable = 0.5*k_cable*D^2;
end

== matlab function Form_Finding_Simulink/24 cables/cable 3--6 ==
  data: out_i output; E_cable output; out_j output; k_cable input; l_cable input; xi input; xj input
function [out_i, E_cable, out_j]= cable(k_cable, l_cable,xi,xj)
% Node distance
dist = norm(xi-xj);

% Difference of node distance with the cable rest length
D = dist-l_cable;

% If the cable is in tension, then the force is calculated. When the cable is slack, the force is zero 
if  dist-l_cable >= 0
    D = dist-l_cable;
elseif dist-l_cable < 0
    D = 0;
end

% Forces on end nodes
out_i = k_cable*D*(xj-xi)/dist;
out_j = -k_cable*D*(xj-xi)/dist;

% Potential energy stored in the cable
E_cable = 0.5*k_cable*D^2;
end

== matlab function Form_Finding_Simulink/24 cables/cable 2--7 ==
  data: out_i output; E_cable output; out_j output; k_cable input; l_cable input; xi input; xj input
function [out_i, E_cable, out_j]= cable(k_cable, l_cable,xi,xj)
% Node distance
dist = norm(xi-xj);

% Difference of node distance with the cable rest length
D = dist-l_cable;

% If the cable is in tension, then the force is calculated. When the cable is slack, the force is zero 
if  dist-l_cable >= 0
    D = dist-l_cable;
elseif dist-l_cable < 0
    D = 0;
end

% Forces on end nodes
out_i = k_cable*D*(xj-xi)/dist;
out_j = -k_cable*D*(xj-xi)/dist;

% Potential energy stored in the cable
E_cable = 0.5*k_cable*D^2;
end

== matlab function Form_Finding_Simulink/24 cables/cable 3--8 ==
  data: out_i output; E_cable output; out_j output; k_cable input; l_cable input; xi input; xj input
function [out_i, E_cable, out_j]= cable(k_cable, l_cable,xi,xj)
% Node distance
dist = norm(xi-xj);

% Difference of node distance with the cable rest length
D = dist-l_cable;

% If the cable is in tension, then the force is calculated. When the cable is slack, the force is zero 
if  dist-l_cable >= 0
    D = dist-l_cable;
elseif dist-l_cable < 0
    D = 0;
end

% Forces on end nodes
out_i = k_cable*D*(xj-xi)/dist;
out_j = -k_cable*D*(xj-xi)/dist;

% Potential energy stored in the cable
E_cable = 0.5*k_cable*D^2;
end

== matlab function Form_Finding_Simulink/24 cables/cable 8--12 ==
  data: out_i output; E_cable output; out_j output; k_cable input; l_cable input; xi input; xj input
function [out_i, E_cable, out_j]= cable(k_cable, l_cable,xi,xj)
% Node distance
dist = norm(xi-xj);

% Difference of node distance with the cable rest length
D = dist-l_cable;

% If the cable is in tension, then the force is calculated. When the cable is slack, the force is zero 
if  dist-l_cable >= 0
    D = dist-l_cable;
elseif dist-l_cable < 0
    D = 0;
end

% Forces on end nodes
out_i = k_cable*D*(xj-xi)/dist;
out_j = -k_cable*D*(xj-xi)/dist;

% Potential energy stored in the cable
E_cable = 0.5*k_cable*D^2;
end

== matlab function Form_Finding_Simulink/24 cables/cable 7--11 ==
  data: out_i output; E_cable output; out_j output; k_cable input; l_cable input; xi input; xj input
function [out_i, E_cable, out_j]= cable(k_cable, l_cable,xi,xj)
% Node distance
dist = norm(xi-xj);

% Difference of node distance with the cable rest length
D = dist-l_cable;

% If the cable is in tension, then the force is calculated. When the cable is slack, the force is zero 
if  dist-l_cable >= 0
    D = dist-l_cable;
elseif dist-l_cable < 0
    D = 0;
end

% Forces on end nodes
out_i = k_cable*D*(xj-xi)/dist;
out_j = -k_cable*D*(xj-xi)/dist;

% Potential energy stored in the cable
E_cable = 0.5*k_cable*D^2;
end

== matlab function Form_Finding_Simulink/24 cables/cable 1--3 ==
  data: out_i output; E_cable output; out_j output; k_cable input; l_cable input; xi input; xj input
function [out_i, E_cable, out_j]= cable(k_cable, l_cable,xi,xj)
% Node distance
dist = norm(xi-xj);

% Difference of node distance with the cable rest length
D = dist-l_cable;

% If the cable is in tension, then the force is calculated. When the cable is slack, the force is zero 
if  dist-l_cable >= 0
    D = dist-l_cable;
elseif dist-l_cable < 0
    D = 0;
end

% Forces on end nodes
out_i = k_cable*D*(xj-xi)/dist;
out_j = -k_cable*D*(xj-xi)/dist;

% Potential energy stored in the cable
E_cable = 0.5*k_cable*D^2;
end

== matlab function Form_Finding_Simulink/24 cables/cable 9--10 ==
  data: out_i output; E_cable output; out_j output; k_cable input; l_cable input; xi input; xj input
function [out_i, E_cable, out_j]= cable(k_cable, l_cable,xi,xj)
% Node distance
dist = norm(xi-xj);

% Difference of node distance with the cable rest length
D = dist-l_cable;

% If the cable is in tension, then the force is calculated. When the cable is slack, the force is zero 
if  dist-l_cable >= 0
    D = dist-l_cable;
elseif dist-l_cable < 0
    D = 0;
end

% Forces on end nodes
out_i = k_cable*D*(xj-xi)/dist;
out_j = -k_cable*D*(xj-xi)/dist;

% Potential energy stored in the cable
E_cable = 0.5*k_cable*D^2;
end

== matlab function Form_Finding_Simulink/24 cables/cable 10--12 ==
  data: out_i output; E_cable output; out_j output; k_cable input; l_cable input; xi input; xj input
function [out_i, E_cable, out_j]= cable(k_cable, l_cable,xi,xj)
% Node distance
dist = norm(xi-xj);

% Difference of node distance with the cable rest length
D = dist-l_cable;

% If the cable is in tension, then the force is calculated. When the cable is slack, the force is zero 
if  dist-l_cable >= 0
    D = dist-l_cable;
elseif dist-l_cable < 0
    D = 0;
end

% Forces on end nodes
out_i = k_cable*D*(xj-xi)/dist;
out_j = -k_cable*D*(xj-xi)/dist;

% Potential energy stored in the cable
E_cable = 0.5*k_cable*D^2;
end

== matlab function Form_Finding_Simulink/24 cables/cable 10--11 ==
  data: out_i output; E_cable output; out_j output; k_cable input; l_cable input; xi input; xj input
function [out_i, E_cable, out_j]= cable(k_cable, l_cable,xi,xj)
% Node distance
dist = norm(xi-xj);

% Difference of node distance with the cable rest length
D = dist-l_cable;

% If the cable is in tension, then the force is calculated. When the cable is slack, the force is zero 
if  dist-l_cable >= 0
    D = dist-l_cable;
elseif dist-l_cable < 0
    D = 0;
end

% Forces on end nodes
out_i = k_cable*D*(xj-xi)/dist;
out_j = -k_cable*D*(xj-xi)/dist;

% Potential energy stored in the cable
E_cable = 0.5*k_cable*D^2;
end

== matlab function Form_Finding_Simulink/24 cables/cable 11--12 ==
  data: out_i output; E_cable output; out_j output; k_cable input; l_cable input; xi input; xj input
function [out_i, E_cable, out_j]= cable(k_cable, l_cable,xi,xj)
% Node distance
dist = norm(xi-xj);

% Difference of node distance with the cable rest length
D = dist-l_cable;

% If the cable is in tension, then the force is calculated. When the cable is slack, the force is zero 
if  dist-l_cable >= 0
    D = dist-l_cable;
elseif dist-l_cable < 0
    D = 0;
end

% Forces on end nodes
out_i = k_cable*D*(xj-xi)/dist;
out_j = -k_cable*D*(xj-xi)/dist;

% Potential energy stored in the cable
E_cable = 0.5*k_cable*D^2;
end

== matlab function Form_Finding_Simulink/24 cables/cable 5--8 ==
  data: out_i output; E_cable output; out_j output; k_cable input; l_cable input; xi input; xj input
function [out_i, E_cable, out_j]= cable(k_cable, l_cable,xi,xj)
% Node distance
dist = norm(xi-xj);

% Difference of node distance with the cable rest length
D = dist-l_cable;

% If the cable is in tension, then the force is calculated. When the cable is slack, the force is zero 
if  dist-l_cable >= 0
    D = dist-l_cable;
elseif dist-l_cable < 0
    D = 0;
end

% Forces on end nodes
out_i = k_cable*D*(xj-xi)/dist;
out_j = -k_cable*D*(xj-xi)/dist;

% Potential energy stored in the cable
E_cable = 0.5*k_cable*D^2;
end

== matlab function Form_Finding_Simulink/24 cables/cable 5--7 ==
  data: out_i output; E_cable output; out_j output; k_cable input; l_cable input; xi input; xj input
function [out_i, E_cable, out_j]= cable(k_cable, l_cable,xi,xj)
% Node distance
dist = norm(xi-xj);

% Difference of node distance with the cable rest length
D = dist-l_cable;

% If the cable is in tension, then the force is calculated. When the cable is slack, the force is zero 
if  dist-l_cable >= 0
    D = dist-l_cable;
elseif dist-l_cable < 0
    D = 0;
end

% Forces on end nodes
out_i = k_cable*D*(xj-xi)/dist;
out_j = -k_cable*D*(xj-xi)/dist;

% Potential energy stored in the cable
E_cable = 0.5*k_cable*D^2;
end

== matlab function Form_Finding_Simulink/24 cables/cable 5--12 ==
  data: out_i output; E_cable output; out_j output; k_cable input; l_cable input; xi input; xj input
function [out_i, E_cable, out_j]= cable(k_cable, l_cable,xi,xj)
% Node distance
dist = norm(xi-xj);

% Difference of node distance with the cable rest length
D = dist-l_cable;

% If the cable is in tension, then the force is calculated. When the cable is slack, the force is zero 
if  dist-l_cable >= 0
    D = dist-l_cable;
elseif dist-l_cable < 0
    D = 0;
end

% Forces on end nodes
out_i = k_cable*D*(xj-xi)/dist;
out_j = -k_cable*D*(xj-xi)/dist;

% Potential energy stored in the cable
E_cable = 0.5*k_cable*D^2;
end

== matlab function Form_Finding_Simulink/24 cables/cable 6--9 ==
  data: out_i output; E_cable output; out_j output; k_cable input; l_cable input; xi input; xj input
function [out_i, E_cable, out_j]= cable(k_cable, l_cable,xi,xj)
% Node distance
dist = norm(xi-xj);

% Difference of node distance with the cable rest length
D = dist-l_cable;

% If the cable is in tension, then the force is calculated. When the cable is slack, the force is zero 
if  dist-l_cable >= 0
    D = dist-l_cable;
elseif dist-l_cable < 0
    D = 0;
end

% Forces on end nodes
out_i = k_cable*D*(xj-xi)/dist;
out_j = -k_cable*D*(xj-xi)/dist;

% Potential energy stored in the cable
E_cable = 0.5*k_cable*D^2;
end

== matlab function Form_Finding_Simulink/24 cables/cable 6--8 ==
  data: out_i output; E_cable output; out_j output; k_cable input; l_cable input; xi input; xj input
function [out_i, E_cable, out_j]= cable(k_cable, l_cable,xi,xj)
% Node distance
dist = norm(xi-xj);

% Difference of node distance with the cable rest length
D = dist-l_cable;

% If the cable is in tension, then the force is calculated. When the cable is slack, the force is zero 
if  dist-l_cable >= 0
    D = dist-l_cable;
elseif dist-l_cable < 0
    D = 0;
end

% Forces on end nodes
out_i = k_cable*D*(xj-xi)/dist;
out_j = -k_cable*D*(xj-xi)/dist;

% Potential energy stored in the cable
E_cable = 0.5*k_cable*D^2;
end

== matlab function Form_Finding_Simulink/24 cables/cable 6--10 ==
  data: out_i output; E_cable output; out_j output; k_cable input; l_cable input; xi input; xj input
function [out_i, E_cable, out_j]= cable(k_cable, l_cable,xi,xj)
% Node distance
dist = norm(xi-xj);

% Difference of node distance with the cable rest length
D = dist-l_cable;

% If the cable is in tension, then the force is calculated. When the cable is slack, the force is zero 
if  dist-l_cable >= 0
    D = dist-l_cable;
elseif dist-l_cable < 0
    D = 0;
end

% Forces on end nodes
out_i = k_cable*D*(xj-xi)/dist;
out_j = -k_cable*D*(xj-xi)/dist;

% Potential energy stored in the cable
E_cable = 0.5*k_cable*D^2;
end

== matlab function Form_Finding_Simulink/24 cables/cable 1--2 ==
  data: out_i output; E_cable output; out_j output; k_cable input; l_cable input; xi input; xj input
function [out_i, E_cable, out_j]= cable(k_cable, l_cable,xi,xj)
% Node distance
dist = norm(xi-xj);

% Difference of node distance with the cable rest length
D = dist-l_cable;

% If the cable is in tension, then the force is calculated. When the cable is slack, the force is zero 
if  dist-l_cable >= 0
    D = dist-l_cable;
elseif dist-l_cable < 0
    D = 0;
end

% Forces on end nodes
out_i = k_cable*D*(xj-xi)/dist;
out_j = -k_cable*D*(xj-xi)/dist;

% Potential energy stored in the cable
E_cable = 0.5*k_cable*D^2;
end

== matlab function Form_Finding_Simulink/12 nodes /node  6/node 6 constrain1 ==
  data: control_out output; control_in input
function control_out = node6_control(control_in)

control_out = [control_in(1);control_in(2);0];

end

== matlab function Form_Finding_Simulink/6 joints/Joint bar 2--8 ==
  data: xi input; alpha output; xj input; xk input; l input; x_joint output
function [alpha, x_joint]  = angle(xi, xj, xk, l)
%% Calculating the angle
d = norm(xi - xj); % Nodal distance
mag = (l^2-2*d^2)/l^2; % Term inside the inverse cosine to calculate the angle
alpha = acos(mag); % Angle of the joint

%% Plotting the Joint
% Distance from axis
d = l/2*cos(alpha/2);

% Vectors used for determination of the normal vector
nxi = transpose(xi);
nxj = transpose(xj);
nxk = transpose(xk);

% Normal vector of a plane created by a set of 2 parallel bars
normal = cross(nxi-nxj, nxi-nxk);
N = normal/norm(normal);

% Vector along the line between bar-connected nodes
x = nxj - nxi;
X = x/norm(x);

% Vector pointing outwards 
V = rotVec(X,N,-90);

% Position vector of the joint, to be used for plotting
x_joint = transpose(d*V + (nxj+nxi)/2);

end

== matlab function Form_Finding_Simulink/6 joints/Force bar 2--8 ==
  data: torsion_i output; torsion_j output; xi input; xj input; m input; k_joint input; alpha input; l_bar input; a_joint input; g input
function [torsion_i, torsion_j]= Force(xi, xj, m, k_joint, alpha, l_bar, a_joint, g)
% Node distance
dist = norm(xj-xi);

% Force exerted by the joint at the end node. The force is zero when the
% deflection angle is larger than a_joint
if alpha < a_joint
    F_torsion = 1/2 * k_joint * (a_joint - alpha) / (cos(alpha/2)*l_bar/2);
else
    F_torsion = 0;
end

% Gravity
Fg_j = m*g/2;

% Calculation of the two parts of the torsion
torsion_i = F_torsion *(xi-xj)/dist + Fg_j;
torsion_j = F_torsion *(xj-xi)/dist + Fg_j;

end

== matlab function Form_Finding_Simulink/6 joints/Angle bar 3--9 ==
  data: xi input; alpha output; xj input; xk input; l input; x_joint output
function [alpha, x_joint]  = angle(xi, xj, xk, l)
%% Calculating the angle
d = norm(xi - xj); % Nodal distance
mag = (l^2-2*d^2)/l^2; % Term inside the inverse cosine to calculate the angle
alpha = acos(mag); % Angle of the joint

%% Plotting the Joint
% Distance from axis
d = l/2*cos(alpha/2);

% Vectors used for determination of the normal vector
nxi = transpose(xi);
nxj = transpose(xj);
nxk = transpose(xk);

% Normal vector of a plane created by a set of 2 parallel bars
normal = cross(nxi-nxj, nxi-nxk);
N = normal/norm(normal);

% Vector along the line between bar-connected nodes
x = nxj - nxi;
X = x/norm(x);

% Vector pointing outwards 
V = rotVec(X,N,-90);

% Position vector of the joint, to be used for plotting
x_joint = transpose(d*V + (nxj+nxi)/2);

end

== matlab function Form_Finding_Simulink/6 joints/Force bar 3--9 ==
  data: F_end_node_1 output; F_end_node_2 output; xi input; x_joint input; xj input; m input; k_joint input; alpha input; l_bar input; a_joint input; g input
function [F_end_node_1, F_end_node_2] = Force(xi,x_joint, xj, m, k_joint, alpha, l_bar, a_joint, g)
% Unit vectors in the direction of the individual bar sections of the leg
unit1 = (x_joint-xi)/norm(x_joint-xi);
unit2 = (xj-x_joint)/norm(xj-x_joint);

% Angles of these bar sections with the ground
theta1 = asin(unit1(3)); 
theta2 = asin(unit2(3));

% Node distance
dist = norm(xj-xi);

% Force exerted by the joint at the end node. The force is zero when the
% deflection angle is larger than a_joint
if alpha < a_joint
    F_torsion = 1/2 * k_joint * (a_joint - alpha) / (cos(alpha/2)*l_bar/2);
else
    F_torsion = 0;
end

% Special case of gravitational force
Fg_joint = m*g/2*cos(theta1);
Fg_j = Fg_joint*sin(theta2) + m*g/2;

% Calculation of the two parts of the torsion
F_end_node_1 = F_torsion *(xi-xj)/dist;
F_end_node_2 = F_torsion *(xj-xi)/dist + Fg_j;

end

== matlab function Form_Finding_Simulink/6 joints/Joint bar 4--10 ==
  data: xi input; alpha output; xj input; xk input; l input; x_joint output
function [alpha, x_joint]  = angle(xi, xj, xk, l)
%% Calculating the angle
d = norm(xi - xj); % Nodal distance
mag = (l^2-2*d^2)/l^2; % Term inside the inverse cosine to calculate the angle
alpha = acos(mag); % Angle of the joint

%% Plotting the Joint
% Distance from axis
d = l/2*cos(alpha/2);

% Vectors used for determination of the normal vector
nxi = transpose(xi);
nxj = transpose(xj);
nxk = transpose(xk);

% Normal vector of a plane created by a set of 2 parallel bars
normal = cross(nxi-nxj, nxi-nxk);
N = normal/norm(normal);

% Vector along the line between bar-connected nodes
x = nxj - nxi;
X = x/norm(x);

% Vector pointing outwards 
V = rotVec(X,N,-90);

% Position vector of the joint, to be used for plotting
x_joint = transpose(d*V + (nxj+nxi)/2);

end

== matlab function Form_Finding_Simulink/6 joints/Force bar 4--10 ==
  data: torsion_i output; torsion_j output; xi input; xj input; m input; k_joint input; alpha input; l_bar input; a_joint input; g input
function [torsion_i, torsion_j]= Force(xi, xj, m, k_joint, alpha, l_bar, a_joint,g)
% Node distance
dist = norm(xj-xi);

% Force exerted by the joint at the end node. The force is zero when the
% deflection angle is larger than a_joint
if alpha < a_joint
    F_torsion = 1/2 * k_joint * (a_joint - alpha) / (cos(alpha/2)*l_bar/2);
else
    F_torsion = 0;
end

% Gravity
Fg_j = m*g/2;

% Calculation of the two parts of the torsion
torsion_i = F_torsion *(xi-xj)/dist + Fg_j;
torsion_j = F_torsion *(xj-xi)/dist + Fg_j;

end

== matlab function Form_Finding_Simulink/6 joints/Joint bar 5--11 ==
  data: xi input; alpha output; xj input; xk input; l input; x_joint output
function [alpha, x_joint]  = angle(xi, xj, xk, l)
%% Calculating the angle
d = norm(xi - xj); % Nodal distance
mag = (l^2-2*d^2)/l^2; % Term inside the inverse cosine to calculate the angle
alpha = acos(mag); % Angle of the joint

%% Plotting the Joint
% Distance from axis
d = l/2*cos(alpha/2);

% Vectors used for determination of the normal vector
nxi = transpose(xi);
nxj = transpose(xj);
nxk = transpose(xk);

% Normal vector of a plane created by a set of 2 parallel bars
normal = cross(nxi-nxj, nxi-nxk);
N = normal/norm(normal);

% Vector along the line between bar-connected nodes
x = nxj - nxi;
X = x/norm(x);

% Vector pointing outwards 
V = rotVec(X,N,-90);

% Position vector of the joint, to be used for plotting
x_joint = transpose(d*V + (nxj+nxi)/2);

end

== matlab function Form_Finding_Simulink/6 joints/Force bar 5--11 ==
  data: torsion_i output; torsion_j output; xi input; xj input; m input; k_joint input; alpha input; l_bar input; a_joint input; g input
function [torsion_i, torsion_j]= Force(xi, xj, m, k_joint, alpha, l_bar, a_joint,g)
% Node distance
dist = norm(xj-xi);

% Force exerted by the joint at the end node. The force is zero when the
% deflection angle is larger than a_joint
if alpha < a_joint
    F_torsion = 1/2 * k_joint * (a_joint - alpha) / (cos(alpha/2)*l_bar/2);
else
    F_torsion = 0;
end

% Gravity
Fg_j = m*g/2;

% Calculation of the two parts of the torsion
torsion_i = F_torsion *(xi-xj)/dist + Fg_j;
torsion_j = F_torsion *(xj-xi)/dist + Fg_j;

end
